simulink model "simpleMicrogrid_v3_0_18a"  (R2018a)
settings: Solver=VariableStepAuto  StartTime=0.0  StopTime=30  RelTol=1e-3
undefined symbols (not defined in the file or in its folder): Ion, Lithium
libraries: simulink x21, spsSeriesRLCBranchLib x13, spsIdealSwitchLib x10, spsMosfetLib x8, spsPWMGeneratorDCDCLib x6, spsVoltageMeasurementLib x5, spsThreePhaseSeriesRLCLoadLib x3, spsThreePhaseSeriesRLCBranchLib x3, spsThreePhaseDynamicLoadLib x3, spsGroundLib x2, spsThreePhaseVIMeasurementLib x2, spsUniversalBridgeLib x2
(part 2 of 2)

== system simpleMicrogrid_v3_0_18a/Power Equation Wind Turbine (PQ Model)1/Wind Turbine Power Equation/Wind Turbine Properties ==
  Wind (m/s) : Inport
  Compare To Constant : simulink/Logic and Bit Operations/Compare To Constant  relop=<  const=Umin  OutDataTypeStr=boolean
  Compare To Constant1 : simulink/Logic and Bit Operations/Compare To Constant  relop=>  const=Umax  OutDataTypeStr=boolean
  Compare To Constant2 : simulink/Logic and Bit Operations/Compare To Constant  relop=<  const=Unom  OutDataTypeStr=boolean
  Logical Operator : Logic  Operator=OR  AllPortsSameDT=off  OutDataTypeStr=boolean
  Max Power : Constant  Value=Pnom
  No Power : Constant  Value=0
  Properties : Subsystem
  Switch : Switch  Criteria=u2 ~= 0  ZeroCross=off
  Switch1 : Switch  Criteria=u2 ~= 0  ZeroCross=off
  Pwind : Outport  VectorParamsAs1DForOutWhenUnconnected=off
  wires:
  Compare To Constant/1 -> Logical Operator/1
  Switch/1 -> Pwind/1
  Logical Operator/1 -> Switch/2
  Wind (m/s)/1 -> Compare To Constant2/1, Properties/1(In1), Compare To Constant1/1, Compare To Constant/1
  Max Power/1 -> Switch1/3
  Switch1/1 -> Switch/3
  No Power/1 -> Switch/1
  Compare To Constant1/1 -> Logical Operator/2
  Compare To Constant2/1 -> Switch1/2
  Properties/1(Out1) -> Switch1/1

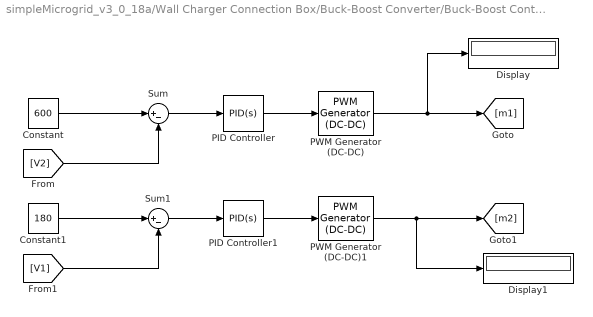
== system simpleMicrogrid_v3_0_18a/Wall Charger Connection Box/Buck-Boost Converter/Buck-Boost Controller ==
  Constant : Constant  Value=600
  Constant1 : Constant  Value=180
  Display : Display
  Display1 : Display
  PID Controller : simulink/Continuous/PID Controller  Controller=PID  Form=Parallel  TimeDomain=Continuous-time  SampleTime=-1  IntegratorMethod=Forward Euler  ControllerParametersSource=internal  P=0  I=7  D=0  UseFilter=on  N=100  TunerSelectOption=Transfer Function Based (PID Tuner App)  InitialConditionSource=internal  InitialConditionForIntegrator=0  InitialConditionForFilter=0  DifferentiatorICPrevScaledInput=0  ExternalReset=none  TrackingMode=off  Kt=1  LimitOutput=off  UpperSaturationLimit=inf  LowerSaturationLimit=-inf  LinearizeAsGain=on  AntiWindupMode=none  Kb=1  POutMin=[]  POutMax=[]  IOutMin=[]  IOutMax=[]  DOutMin=[]  DOutMax=[]  NOutMin=[]  NOutMax=[]  SumOutMin=[]  SumOutMax=[]  SaturationOutMin=[]  SaturationOutMax=[]  PParamMin=[]  PParamMax=[]  IParamMin=[]  IParamMax=[]  DParamMin=[]  DParamMax=[]  NParamMin=[]  NParamMax=[]  KbParamMin=[]  KbParamMax=[]  KtParamMin=[]  KtParamMax=[]  KbOutMin=[]  KbOutMax=[]  KtOutMin=[]  KtOutMax=[]  IntegratorOutMin=[]  IntegratorOutMax=[]  FilterOutMin=[]  FilterOutMax=[]  SumI1OutMin=[]  SumI1OutMax=[]  SumI2OutMin=[]  SumI2OutMax=[]  SumI3OutMin=[]  SumI3OutMax=[]  SumDOutMin=[]  SumDOutMax=[]  DifferentiatorOutMin=[]  DifferentiatorOutMax=[]  FilterDiffOutCoefMin=[]  FilterDiffOutCoefMax=[]  ReciprocalOutMin=[]  ReciprocalOutMax=[]  SumDenOutMin=[]  SumDenOutMax=[]  SumNumOutMin=[]  SumNumOutMax=[]  DivideOutMin=[]  DivideOutMax=[]  IntegratorContinuousStateAttributes=''  IntegratorStateMustResolveToSignalObject=off  IntegratorRTWStateStorageClass=Auto  FilterContinuousStateAttributes=''  FilterStateMustResolveToSignalObject=off  FilterRTWStateStorageClass=Auto
  PID Controller1 : simulink/Continuous/PID Controller  Controller=PID  Form=Parallel  TimeDomain=Continuous-time  SampleTime=-1  IntegratorMethod=Forward Euler  ControllerParametersSource=internal  P=0  I=7  D=0  UseFilter=on  N=100  TunerSelectOption=Transfer Function Based (PID Tuner App)  InitialConditionSource=internal  InitialConditionForIntegrator=0  InitialConditionForFilter=0  DifferentiatorICPrevScaledInput=0  ExternalReset=none  TrackingMode=off  Kt=1  LimitOutput=off  UpperSaturationLimit=inf  LowerSaturationLimit=-inf  LinearizeAsGain=on  AntiWindupMode=none  Kb=1  POutMin=[]  POutMax=[]  IOutMin=[]  IOutMax=[]  DOutMin=[]  DOutMax=[]  NOutMin=[]  NOutMax=[]  SumOutMin=[]  SumOutMax=[]  SaturationOutMin=[]  SaturationOutMax=[]  PParamMin=[]  PParamMax=[]  IParamMin=[]  IParamMax=[]  DParamMin=[]  DParamMax=[]  NParamMin=[]  NParamMax=[]  KbParamMin=[]  KbParamMax=[]  KtParamMin=[]  KtParamMax=[]  KbOutMin=[]  KbOutMax=[]  KtOutMin=[]  KtOutMax=[]  IntegratorOutMin=[]  IntegratorOutMax=[]  FilterOutMin=[]  FilterOutMax=[]  SumI1OutMin=[]  SumI1OutMax=[]  SumI2OutMin=[]  SumI2OutMax=[]  SumI3OutMin=[]  SumI3OutMax=[]  SumDOutMin=[]  SumDOutMax=[]  DifferentiatorOutMin=[]  DifferentiatorOutMax=[]  FilterDiffOutCoefMin=[]  FilterDiffOutCoefMax=[]  ReciprocalOutMin=[]  ReciprocalOutMax=[]  SumDenOutMin=[]  SumDenOutMax=[]  SumNumOutMin=[]  SumNumOutMax=[]  DivideOutMin=[]  DivideOutMax=[]  IntegratorContinuousStateAttributes=''  IntegratorStateMustResolveToSignalObject=off  IntegratorRTWStateStorageClass=Auto  FilterContinuousStateAttributes=''  FilterStateMustResolveToSignalObject=off  FilterRTWStateStorageClass=Auto
  PWM Generator (DC-DC) : spsPWMGeneratorDCDCLib/PWM Generator (DC-DC)  Fsw=5000  Ts=0
  PWM Generator (DC-DC)1 : spsPWMGeneratorDCDCLib/PWM Generator (DC-DC)  Fsw=5000  Ts=0
  Sum : Sum  Inputs=|+-
  Sum1 : Sum  Inputs=|+-
  wires:
  Constant/1 -> Sum/1
  [V2] -> Sum/2
  Sum/1 -> PID Controller/1
  Sum1/1 -> PID Controller1/1
  Constant1/1 -> Sum1/1
  [V1] -> Sum1/2
  PID Controller/1 -> PWM Generator (DC-DC)/1
  PID Controller1/1 -> PWM Generator (DC-DC)1/1
  PWM Generator (DC-DC)/1 -> Display/1, [m1]
  PWM Generator (DC-DC)1/1 -> Display1/1, [m2]

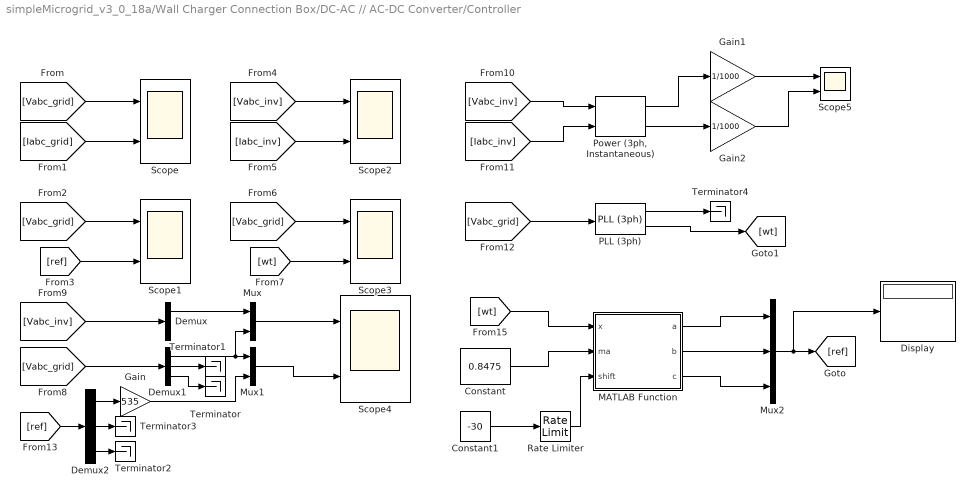
== system simpleMicrogrid_v3_0_18a/Wall Charger Connection Box/DC-AC // AC-DC Converter/Controller ==
  Constant : Constant  Value=0.8475
  Constant1 : Constant  Value=-30
  Demux : Demux  Outputs=3
  Demux1 : Demux  Outputs=3
  Demux2 : Demux  Outputs=3
  Display : Display
  Gain : Gain  Gain=535
  Gain1 : Gain  Gain=1/1000
  Gain2 : Gain  Gain=1/1000
  MATLAB Function : MATLAB Function  TreatAsAtomicUnit=on
  Mux : Mux  Inputs=2
  Mux1 : Mux  Inputs=2
  Mux2 : Mux  Inputs=3
  PLL (3ph) : spsPLL3phLib/PLL (3ph)  Fmin=45  Par_Init=[0, 50]  ParK=[180, 3200, 1]  TcD=1e-4  MaxRateChangeFreq=12  FilterCutOffFreq=25  Ts=2.02e-6  AGC=on
  "Power (3ph, Instantaneous)" : spsPower3phInstantaneousLib/Power (3ph, Instantaneous)
  Rate Limiter : RateLimiter  SampleTimeMode=inherited
  Scope{,1..5} (6 alike) : Scope  NumInputPorts=2
  Terminator{,1..4} (5 alike) : Terminator
  wires:
  [Vabc_grid] -> Scope/1
  [Iabc_grid] -> Scope/2
  [ref] -> Scope1/2
  [Vabc_grid] -> Scope1/1
  [Iabc_inv] -> Scope2/2
  [Vabc_inv] -> Scope2/1
  [wt] -> Scope3/2
  [Vabc_grid] -> Scope3/1
  [Vabc_inv] -> Demux/1
  Demux/1 -> Mux/1
  [Vabc_grid] -> Demux1/1
  Demux1/1 -> Mux/2, Mux1/1
  Demux1/2 -> Terminator1/1
  Demux1/3 -> Terminator/1
  Mux/1 -> Scope4/1
  Mux1/1 -> Scope4/2
  [ref] -> Demux2/1
  Demux2/2 -> Terminator3/1
  Demux2/3 -> Terminator2/1
  Demux2/1 -> Gain/1
  Gain/1 -> Mux1/2
  Constant1/1 -> Rate Limiter/1
  Mux2/1 -> Display/1, [ref]
  [Vabc_inv] -> "Power (3ph, Instantaneous)"/1
  [Iabc_inv] -> "Power (3ph, Instantaneous)"/2
  "Power (3ph, Instantaneous)"/1 -> Gain1/1
  Gain1/1 -> Scope5/1
  "Power (3ph, Instantaneous)"/2 -> Gain2/1
  Gain2/1 -> Scope5/2
  [Vabc_grid] -> PLL (3ph)/1
  PLL (3ph)/1 -> Terminator4/1
  PLL (3ph)/2 -> [wt]
  [wt] -> MATLAB Function/1(x)
  Constant/1 -> MATLAB Function/2(ma)
  Rate Limiter/1 -> MATLAB Function/3(shift)
  MATLAB Function/2(b) -> Mux2/2
  MATLAB Function/1(a) -> Mux2/1
  MATLAB Function/3(c) -> Mux2/3

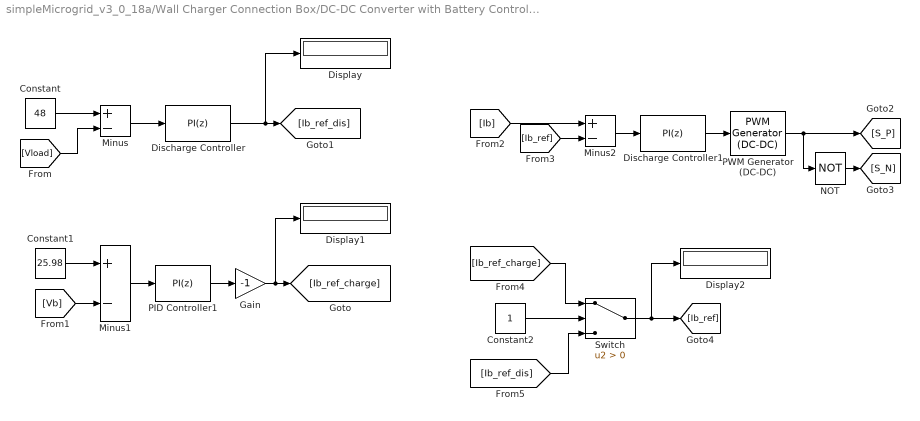
== system simpleMicrogrid_v3_0_18a/Wall Charger Connection Box/DC-DC Converter with Battery Controller/Battery Controller ==
  Constant : Constant  Value=48
  Constant1 : Constant  Value=25.98
  Constant2 : Constant
  Discharge Controller : simulink/Continuous/PID Controller  Controller=PI  Form=Parallel  TimeDomain=Discrete-time  SampleTime=500e-6  IntegratorMethod=Forward Euler  ControllerParametersSource=internal  P=0.25  I=50  D=0  UseFilter=on  N=100  TunerSelectOption=Transfer Function Based (PID Tuner App)  InitialConditionSource=internal  InitialConditionForIntegrator=0  InitialConditionForFilter=0  DifferentiatorICPrevScaledInput=0  ExternalReset=none  TrackingMode=off  Kt=1  LimitOutput=on  UpperSaturationLimit=22  LowerSaturationLimit=0  LinearizeAsGain=off  AntiWindupMode=none  Kb=1  POutMin=[]  POutMax=[]  IOutMin=[]  IOutMax=[]  DOutMin=[]  DOutMax=[]  NOutMin=[]  NOutMax=[]  SumOutMin=[]  SumOutMax=[]  SaturationOutMin=[]  SaturationOutMax=[]  PParamMin=[]  PParamMax=[]  IParamMin=[]  IParamMax=[]  DParamMin=[]  DParamMax=[]  NParamMin=[]  NParamMax=[]  KbParamMin=[]  KbParamMax=[]  KtParamMin=[]  KtParamMax=[]  KbOutMin=[]  KbOutMax=[]  KtOutMin=[]  KtOutMax=[]  IntegratorOutMin=[]  IntegratorOutMax=[]  FilterOutMin=[]  FilterOutMax=[]  SumI1OutMin=[]  SumI1OutMax=[]  SumI2OutMin=[]  SumI2OutMax=[]  SumI3OutMin=[]  SumI3OutMax=[]  SumDOutMin=[]  SumDOutMax=[]  DifferentiatorOutMin=[]  DifferentiatorOutMax=[]  FilterDiffOutCoefMin=[]  FilterDiffOutCoefMax=[]  ReciprocalOutMin=[]  ReciprocalOutMax=[]  SumDenOutMin=[]  SumDenOutMax=[]  SumNumOutMin=[]  SumNumOutMax=[]  DivideOutMin=[]  DivideOutMax=[]  IntegratorContinuousStateAttributes=''  IntegratorStateMustResolveToSignalObject=off  IntegratorRTWStateStorageClass=Auto  FilterContinuousStateAttributes=''  FilterStateMustResolveToSignalObject=off  FilterRTWStateStorageClass=Auto
  Discharge Controller1 : simulink/Continuous/PID Controller  Controller=PI  Form=Parallel  TimeDomain=Discrete-time  SampleTime=50e-6  IntegratorMethod=Forward Euler  ControllerParametersSource=internal  P=0.005  I=10  D=0  UseFilter=on  N=100  TunerSelectOption=Transfer Function Based (PID Tuner App)  InitialConditionSource=internal  InitialConditionForIntegrator=0.54  InitialConditionForFilter=0  DifferentiatorICPrevScaledInput=0  ExternalReset=none  TrackingMode=off  Kt=1  LimitOutput=on  UpperSaturationLimit=0.95  LowerSaturationLimit=0  LinearizeAsGain=off  AntiWindupMode=none  Kb=1  POutMin=[]  POutMax=[]  IOutMin=[]  IOutMax=[]  DOutMin=[]  DOutMax=[]  NOutMin=[]  NOutMax=[]  SumOutMin=[]  SumOutMax=[]  SaturationOutMin=[]  SaturationOutMax=[]  PParamMin=[]  PParamMax=[]  IParamMin=[]  IParamMax=[]  DParamMin=[]  DParamMax=[]  NParamMin=[]  NParamMax=[]  KbParamMin=[]  KbParamMax=[]  KtParamMin=[]  KtParamMax=[]  KbOutMin=[]  KbOutMax=[]  KtOutMin=[]  KtOutMax=[]  IntegratorOutMin=[]  IntegratorOutMax=[]  FilterOutMin=[]  FilterOutMax=[]  SumI1OutMin=[]  SumI1OutMax=[]  SumI2OutMin=[]  SumI2OutMax=[]  SumI3OutMin=[]  SumI3OutMax=[]  SumDOutMin=[]  SumDOutMax=[]  DifferentiatorOutMin=[]  DifferentiatorOutMax=[]  FilterDiffOutCoefMin=[]  FilterDiffOutCoefMax=[]  ReciprocalOutMin=[]  ReciprocalOutMax=[]  SumDenOutMin=[]  SumDenOutMax=[]  SumNumOutMin=[]  SumNumOutMax=[]  DivideOutMin=[]  DivideOutMax=[]  IntegratorContinuousStateAttributes=''  IntegratorStateMustResolveToSignalObject=off  IntegratorRTWStateStorageClass=Auto  FilterContinuousStateAttributes=''  FilterStateMustResolveToSignalObject=off  FilterRTWStateStorageClass=Auto
  Display : Display
  Display1 : Display
  Display2 : Display
  Gain : Gain  Gain=-1
  Minus : Sum  Inputs=+-
  Minus1 : Sum  Inputs=+-
  Minus2 : Sum  Inputs=+-
  NOT : Logic  Operator=NOT  IconShape=distinctive  AllPortsSameDT=off  OutDataTypeStr=boolean
  PID Controller1 : simulink/Continuous/PID Controller  Controller=PI  Form=Parallel  TimeDomain=Discrete-time  SampleTime=50e-6  IntegratorMethod=Forward Euler  ControllerParametersSource=internal  P=40  I=2000  D=0  UseFilter=on  N=100  TunerSelectOption=Transfer Function Based (PID Tuner App)  InitialConditionSource=internal  InitialConditionForIntegrator=0  InitialConditionForFilter=0  DifferentiatorICPrevScaledInput=0  ExternalReset=none  TrackingMode=off  Kt=1  LimitOutput=on  UpperSaturationLimit=22  LowerSaturationLimit=0  LinearizeAsGain=off  AntiWindupMode=none  Kb=1  POutMin=[]  POutMax=[]  IOutMin=[]  IOutMax=[]  DOutMin=[]  DOutMax=[]  NOutMin=[]  NOutMax=[]  SumOutMin=[]  SumOutMax=[]  SaturationOutMin=[]  SaturationOutMax=[]  PParamMin=[]  PParamMax=[]  IParamMin=[]  IParamMax=[]  DParamMin=[]  DParamMax=[]  NParamMin=[]  NParamMax=[]  KbParamMin=[]  KbParamMax=[]  KtParamMin=[]  KtParamMax=[]  KbOutMin=[]  KbOutMax=[]  KtOutMin=[]  KtOutMax=[]  IntegratorOutMin=[]  IntegratorOutMax=[]  FilterOutMin=[]  FilterOutMax=[]  SumI1OutMin=[]  SumI1OutMax=[]  SumI2OutMin=[]  SumI2OutMax=[]  SumI3OutMin=[]  SumI3OutMax=[]  SumDOutMin=[]  SumDOutMax=[]  DifferentiatorOutMin=[]  DifferentiatorOutMax=[]  FilterDiffOutCoefMin=[]  FilterDiffOutCoefMax=[]  ReciprocalOutMin=[]  ReciprocalOutMax=[]  SumDenOutMin=[]  SumDenOutMax=[]  SumNumOutMin=[]  SumNumOutMax=[]  DivideOutMin=[]  DivideOutMax=[]  IntegratorContinuousStateAttributes=''  IntegratorStateMustResolveToSignalObject=off  IntegratorRTWStateStorageClass=Auto  FilterContinuousStateAttributes=''  FilterStateMustResolveToSignalObject=off  FilterRTWStateStorageClass=Auto
  PWM Generator (DC-DC) : spsPWMGeneratorDCDCLib/PWM Generator (DC-DC)  Fsw=10e3  Ts=5e-6
  Switch : Switch  Criteria=u2 > Threshold
  wires:
  Constant/1 -> Minus/1
  [Vload] -> Minus/2
  [Vb] -> Minus1/2
  Constant1/1 -> Minus1/1
  Gain/1 -> Display1/1, [Ib_ref_charge]
  Minus/1 -> Discharge Controller/1
  Minus1/1 -> PID Controller1/1
  Discharge Controller/1 -> Display/1, [Ib_ref_dis]
  [Ib] -> Minus2/1
  [Ib_ref] -> Minus2/2
  Minus2/1 -> Discharge Controller1/1
  Discharge Controller1/1 -> PWM Generator (DC-DC)/1
  PWM Generator (DC-DC)/1 -> NOT/1, [S_P]
  NOT/1 -> [S_N]
  PID Controller1/1 -> Gain/1
  [Ib_ref_charge] -> Switch/1
  Constant2/1 -> Switch/2
  [Ib_ref_dis] -> Switch/3
  Switch/1 -> Display2/1, [Ib_ref]

== system simpleMicrogrid_v3_0_18a/Power Equation Wind Turbine (PQ Model)/Wind Turbine Power Equation/Wind Turbine Properties/Properties ==
  In1 : Inport
  Air Density : Gain  Gain=rho
  Blade Swept Area (m^2) : Gain  Gain=A
  Gain : Gain  Gain=1/2
  Power Coefficient : Constant  Value=Cp
  "Product " : Product  SaturateOnIntegerOverflow=on  OutDataTypeStr=Inherit: Same as first input
  wind_speed^3 : Fcn  Expr=u(1)^3
  Out1 : Outport  VectorParamsAs1DForOutWhenUnconnected=off
  wires:
  Gain/1 -> Blade Swept Area (m^2)/1
  "Product "/1 -> Out1/1
  Air Density/1 -> Gain/1
  In1/1 -> wind_speed^3/1
  Power Coefficient/1 -> "Product "/2
  wind_speed^3/1 -> Air Density/1
  Blade Swept Area (m^2)/1 -> "Product "/1

== system simpleMicrogrid_v3_0_18a/Power Equation Wind Turbine (PQ Model)1/Wind Turbine Power Equation/Wind Turbine Properties/Properties ==
  In1 : Inport
  Air Density : Gain  Gain=rho
  Blade Swept Area (m^2) : Gain  Gain=A
  Gain : Gain  Gain=1/2
  Power Coefficient : Constant  Value=Cp
  "Product " : Product  SaturateOnIntegerOverflow=on  OutDataTypeStr=Inherit: Same as first input
  wind_speed^3 : Fcn  Expr=u(1)^3
  Out1 : Outport  VectorParamsAs1DForOutWhenUnconnected=off
  wires:
  Gain/1 -> Blade Swept Area (m^2)/1
  "Product "/1 -> Out1/1
  Air Density/1 -> Gain/1
  In1/1 -> wind_speed^3/1
  Power Coefficient/1 -> "Product "/2
  wind_speed^3/1 -> Air Density/1
  Blade Swept Area (m^2)/1 -> "Product "/1

== matlab function simpleMicrogrid_v3_0_18a/Wall Charger Connection Box/DC-AC // AC-DC Converter/Controller/MATLAB Function ==
  data: x input; a output; ma input; shift input; b output; c output
function [a,b,c] = ref_generation(x, ma,shift)
 shift_k=shift*pi/180;
 a=(ma*(sin((x)+shift_k)));
 b=(ma*(sin((x)+shift_k-(2*pi/3))));
 c=(ma*(sin((x)+shift_k+(2*pi/3))));
